simulink model "LaneChangePlanner"  (R2020b)
settings: Solver=FixedStepAuto  StartTime=0.0  StopTime=10.0  RelTol=1e-3
values from neighbouring files (symbols this model uses):
  minDistThreshold = 3.7    [setupscript.m]
  Ts = 0.1    [setupscript.m]
  v0_ego = egoCar.v0    [setupscript.m]
undefined symbols (not defined in the file or in its folder): planningHorizon
settings Model: Creator=The MathWorks, Inc.  LastModifiedBy=Milin
settings OptimizationCC: DefaultParameterBehavior=Inlined  EnhancedBackFolding=on  PassReuseOutputArgsAs=Individual arguments  ZeroExternalMemoryAtStartup=off  ZeroInternalMemoryAtStartup=off  OptimizeBlockOrder=speed  DifferentSizesBufferReuse=on  OptimizationCustomize=off  EfficientTunableParamExpr=on
settings DebuggingCC: ParameterTunabilityLossMsg=error
settings ModelReferenceCC: ModelReferenceNumInstancesAllowed=Single  PropagateVarSize=During execution
settings SFSimCC: MATLABDynamicMemAllocThreshold=0
settings RTWCC: Description=Embedded Coder  SystemTargetFile=ert.tlc  TemplateMakefile=ert_default_tmf
settings CodeAppCC: ForceParamTrailComments=on  IgnoreCustomStorageClasses=off  OperatorAnnotations=on  SimulinkDataObjDesc=on  SFDataObjDesc=on  InsertBlockDesc=on
settings ERTTargetCC: TargetLangStandard=C99 (ISO)  GenerateSampleERTMain=on  SupportVariableSizeSignals=on  InlinedParameterPlacement=NonHierarchical  ERTCustomFileTemplate=example_file_process.tlc

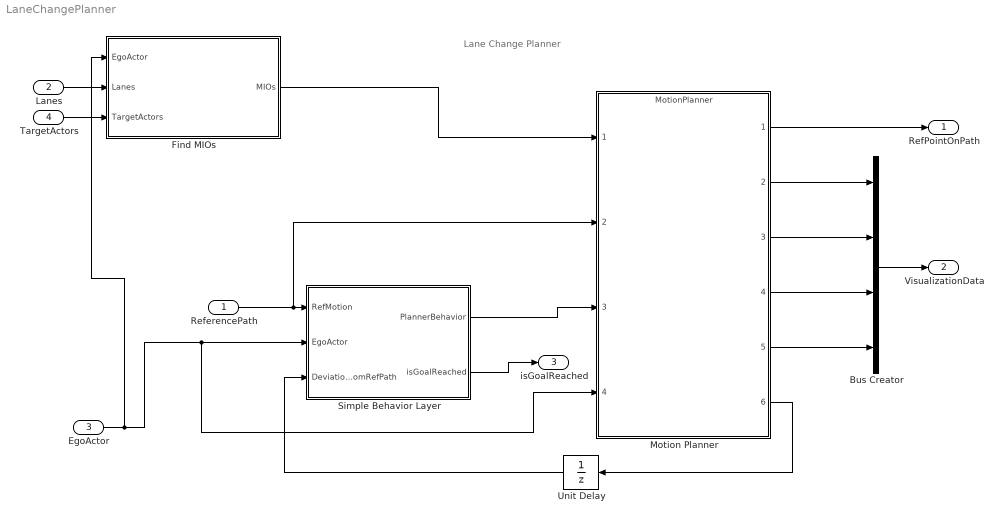
== system LaneChangePlanner ==
  note: Lane Change Planner
  ReferencePath : Inport
  Lanes : Inport  Port=2  OutDataTypeStr=Bus: BusLanes  BusOutputAsStruct=on
  EgoActor : Inport  Port=3  OutDataTypeStr=Bus: BusActors1Actors  BusOutputAsStruct=on
  TargetActors : Inport  Port=4  OutDataTypeStr=Bus: BusActors1  BusOutputAsStruct=on
  Bus Creator : BusCreator  Inputs=4  OutDataTypeStr=Bus: BusPlannerData
  Find MIOs : Subsystem
  Motion Planner : ModelReference  ModelNameDialog=MotionPlanner.slx  SimulationMode=Normal  CodeInterface=Top model  ModelReferenceVersion=1.92
  Simple Behavior Layer : Subsystem
  Unit Delay : UnitDelay  InitialCondition=-1.8000  SampleTime=-1  HasFrameUpgradeWarning=on
  RefPointOnPath : Outport  OutDataTypeStr=Bus: BusRefPointOnPath
  VisualizationData : Outport  Port=2  OutDataTypeStr=Bus: BusPlannerData
  isGoalReached : Outport  Port=3
  wires:
  Unit Delay/1 -> Simple Behavior Layer/3(DeviationFromRefPath)
  Motion Planner/6 -> Unit Delay/1
  Simple Behavior Layer/2(isGoalReached) -> isGoalReached/1
  Motion Planner/5 -> Bus Creator/4
  Bus Creator/1 -> VisualizationData/1
  Motion Planner/3 -> Bus Creator/2
  Motion Planner/4 -> Bus Creator/3
  Motion Planner/2 -> Bus Creator/1
  ReferencePath/1 -> Motion Planner/2, Simple Behavior Layer/1(RefMotion)
  Motion Planner/1 -> RefPointOnPath/1
  EgoActor/1 -> Find MIOs/1(EgoActor), Motion Planner/4, Simple Behavior Layer/2(EgoActor)
  Lanes/1 -> Find MIOs/2(Lanes)
  TargetActors/1 -> Find MIOs/3(TargetActors)
  Simple Behavior Layer/1(PlannerBehavior) -> Motion Planner/3
  Find MIOs/1(MIOs) -> Motion Planner/1

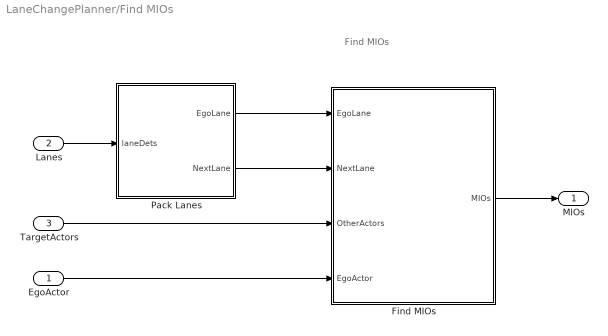
== system LaneChangePlanner/Find MIOs ==
  note: Find MIOs
  EgoActor : Inport
  Lanes : Inport  Port=2
  TargetActors : Inport  Port=3
  Find MIOs : MATLAB Function  TreatAsAtomicUnit=on
  Pack Lanes : MATLAB Function  TreatAsAtomicUnit=on
  MIOs : Outport
  wires:
  Pack Lanes/2(NextLane) -> Find MIOs/2(NextLane)
  Pack Lanes/1(EgoLane) -> Find MIOs/1(EgoLane)
  Lanes/1 -> Pack Lanes/1(laneDets)
  EgoActor/1 -> Find MIOs/4(EgoActor)
  TargetActors/1 -> Find MIOs/3(OtherActors)
  Find MIOs/1(MIOs) -> MIOs/1

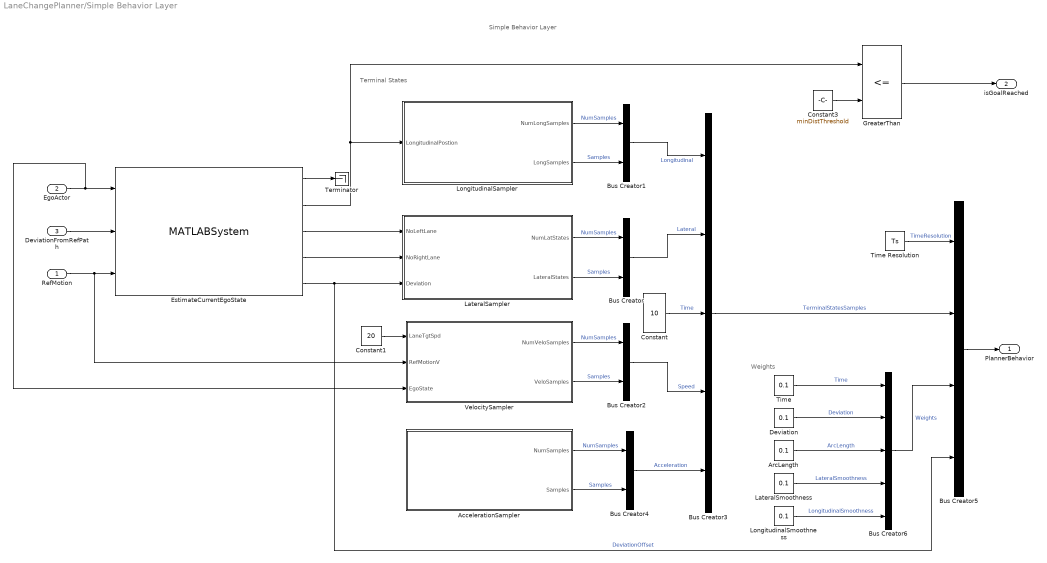
== system LaneChangePlanner/Simple Behavior Layer ==
  note: Weights
  note: Terminal States
  note: Simple Behavior Layer
  RefMotion : Inport
  EgoActor : Inport  Port=2
  DeviationFromRefPath : Inport  Port=3
  AccelerationSampler : Subsystem
  ArcLength : Constant  Value=0.1
  Bus Creator{,1..2,4} (4 alike) : BusCreator  Inputs=2
  Bus Creator3 : BusCreator  Inputs=5
  Bus Creator5 : BusCreator  Inputs=4  OutDataTypeStr=Bus: BusPlannerBehavior  NonVirtualBus=on
  Bus Creator6 : BusCreator  Inputs=5
  Constant : Constant  Value=10
  Constant1 : Constant  Value=20
  Constant3 : Constant  Value=minDistThreshold
  Deviation : Constant  Value=0.1
  EstimateCurrentEgoState : MATLABSystem  System=HelperEstimateCurrentEgoState  LaneWidth=laneWidth  EgoActorID=1  InitialDeviation=initialDeviation  InitialEgoLaneNumber=initialEgoLaneID  LaneType=laneType  SimulateUsing=Code generation
      mask Type: HelperEstimateCurrentEgoState
      mask Display:
      | disp('HelperEstimateCurrentEgoState');
      | port_label('input',1,'EgoActor');
      | port_label('input',2,'LateralDeviation');
      | port_label('input',3,'RefPath');
      | port_label('output',1,'LateralPosition');
      | port_label('output',2,'LongitudinalPosition');
      | port_label('output',3,'NoLeftLane');
      | port_label('output',4,'NoRightLane');
      | port_label('output',5,'DeviationOffset');
  GreaterThan : RelationalOperator  Operator=<=  OutDataTypeStr=boolean  RndMeth=Simplest
  LateralSampler : MATLAB Function  TreatAsAtomicUnit=on
  LateralSmoothness : Constant  Value=0.1
  LongitudinalSampler : MATLAB Function  TreatAsAtomicUnit=on  mask{planningHorizon=planningHorizon}
      mask prompts: planningHorizon "Planning Horizon"
  LongitudinalSmoothness : Constant  Value=0.1
  Terminator : Terminator
  Time : Constant  Value=0.1
  Time Resolution : Constant  Value=Ts
  VelocitySampler : MATLAB Function  TreatAsAtomicUnit=on  mask{egoSetVelocity=v0_ego}
      mask prompts: egoSetVelocity "Ego Set Velocity"
  PlannerBehavior : Outport  OutDataTypeStr=Bus: BusPlannerBehavior
  isGoalReached : Outport  Port=2
  wires:
  GreaterThan/1 -> isGoalReached/1
  VelocitySampler/2(VeloSamples) -> Bus Creator2/2  "Samples"
  RefMotion/1 -> EstimateCurrentEgoState/3, VelocitySampler/2(RefMotionV)
  EgoActor/1 -> EstimateCurrentEgoState/1, VelocitySampler/3(EgoState)
  Constant1/1 -> VelocitySampler/1(LaneTgtSpd)
  VelocitySampler/1(NumVeloSamples) -> Bus Creator2/1  "NumSamples"
  Constant3/1 -> GreaterThan/2
  Constant/1 -> Bus Creator3/3  "Time"
  EstimateCurrentEgoState/4 -> LateralSampler/2(NoRightLane)
  EstimateCurrentEgoState/3 -> LateralSampler/1(NoLeftLane)
  EstimateCurrentEgoState/2 -> GreaterThan/1, LongitudinalSampler/1(LongitudinalPostion)
  LongitudinalSampler/1(NumLongSamples) -> Bus Creator1/1  "NumSamples"
  LongitudinalSampler/2(LongSamples) -> Bus Creator1/2  "Samples"
  Bus Creator1/1 -> Bus Creator3/1  "Longitudinal"
  Bus Creator2/1 -> Bus Creator3/4  "Speed"
  EstimateCurrentEgoState/5 -> Bus Creator5/4, LateralSampler/3(Deviation)  "DeviationOffset"
  Bus Creator/1 -> Bus Creator3/2  "Lateral"
  LateralSampler/2(LateralStates) -> Bus Creator/2  "Samples"
  Bus Creator6/1 -> Bus Creator5/3  "Weights"
  Bus Creator3/1 -> Bus Creator5/2  "TerminalStatesSamples"
  Time Resolution/1 -> Bus Creator5/1  "TimeResolution"
  LongitudinalSmoothness/1 -> Bus Creator6/5  "LongitudinalSmoothness"
  LateralSmoothness/1 -> Bus Creator6/4  "LateralSmoothness"
  ArcLength/1 -> Bus Creator6/3  "ArcLength"
  Deviation/1 -> Bus Creator6/2  "Deviation"
  Time/1 -> Bus Creator6/1  "Time"
  Bus Creator4/1 -> Bus Creator3/5  "Acceleration"
  LateralSampler/1(NumLatStates) -> Bus Creator/1  "NumSamples"
  AccelerationSampler/2(Samples) -> Bus Creator4/2  "Samples"
  AccelerationSampler/1(NumSamples) -> Bus Creator4/1  "NumSamples"
  EstimateCurrentEgoState/1 -> Terminator/1
  Bus Creator5/1 -> PlannerBehavior/1
  DeviationFromRefPath/1 -> EstimateCurrentEgoState/2

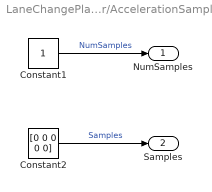
== system LaneChangePlanner/Simple Behavior Layer/AccelerationSampler ==
  Constant1 : Constant
  Constant2 : Constant  Value=[0 0 0 0 0]
  NumSamples : Outport
  Samples : Outport  Port=2
  wires:
  Constant1/1 -> NumSamples/1  "NumSamples"
  Constant2/1 -> Samples/1  "Samples"

== matlab function LaneChangePlanner/Find MIOs/Find MIOs ==
  data: EgoLane input; NextLane input; OtherActors input; EgoActor input; MIOs output Bus: BusMIOs
% Find front/rear MIO (Most Important Object) in the ego lane and front/rear
% MIOs in the left next lane.
function MIOs  = findMIOs( EgoLane, NextLane, OtherActors, EgoActor)

% If lane detection is not available, the ego car is assumed to be located
% in the middle of its lane. The lane width is assumed to be 3.6m, typical
% highway lane width.
laneWidth = 3.6;
halfLaneWidth = laneWidth/2;

% ego left lane detected?
if EgoLane.Left.Strength > 0.01 
    egoLeftLane = [EgoLane.Left.CurvatureDerivative/6,...
        EgoLane.Left.Curvature/2,...
        EgoLane.Left.HeadingAngle,...
        EgoLane.Left.LateralOffset];
else % ego left lane is not available
    egoLeftLane = single([0,0,0,halfLaneWidth]);
end
% ego right lane detected?
if EgoLane.Right.Strength > 0.01  
    egoRightLane = [EgoLane.Right.CurvatureDerivative/6,...
        EgoLane.Right.Curvature/2,...
        EgoLane.Right.HeadingAngle,...
        EgoLane.Right.LateralOffset];
else % ego right lane is not available
    egoRightLane = single([0,0,0,-halfLaneWidth]);    
end
% left next lane detected?
if NextLane.Left.Strength > 0.01 
    nextLeftLane = [NextLane.Left.CurvatureDerivative/6,...
        NextLane.Left.Curvature/2,...
        NextLane.Left.HeadingAngle,...
        NextLane.Left.LateralOffset];
else % left next lane is not available
    nextLeftLane = single([0,0,0,halfLaneWidth+laneWidth]);       
end
% right next lane detected?
if NextLane.Right.Strength > 0.01 
    nextRightLane = [NextLane.Right.CurvatureDerivative/6,...
        NextLane.Right.Curvature/2,...
        NextLane.Right.HeadingAngle,...
        NextLane.Right.LateralOffset];
else % right next lane is not available
    nextRightLane = single([0,0,0,halfLaneWidth+laneWidth]);       
end

% Initialize outputs and parameters
% Far enough forward so that no track is expected to exceed this distance
egoMaxX = cast(500, 'like', EgoActor.Position);
% Far enough forward so that no track is expected to exceed this distance
egoMinX = cast(-500, 'like', EgoActor.Position);  
% Far enough forward so that no track is expected to exceed this distance
leftNextMaxX = cast(500, 'like', EgoActor.Position);  
% Far enough rearward so that no track is expected to exceed this distance
leftNextMinX = cast(-500, 'like', EgoActor.Position);  
% Far enough forward so that no track is expected to exceed this distance
rightNextMaxX = cast(500, 'like', EgoActor.Position); 
% Far enough rearward so that no track is expected to exceed this distance
rightNextMinX = cast(-500, 'like', EgoActor.Position);

% initialize MIOs
EgoFront = struct(...
    'TrackIndex', uint32(0),...
    'Position', double([0 0]'), ...
    'Velocity', double([0 0]'), ...
    'RangeMagnitude', double(2000), ...  % default range = big number (ex. 2000)
    'VelocityMagnitude', double(0), ...
    'TTC', double(100));

EgoRear = struct(...
    'TrackIndex', uint32(0),...
    'Position', double([0 0]'), ...
    'Velocity', double([0 0]'), ...
    'RangeMagnitude', double(0), ...  
    'VelocityMagnitude', double(0), ...
    'TTC', double(0));

LeftFront = struct(...
    'TrackIndex', uint32(0),...
    'Position', double([0 0]'), ...
    'Velocity', double([0 0]'), ...
    'RangeMagnitude', double(0), ...
    'VelocityMagnitude', double(0), ...
    'TTC', double(0));

LeftRear = struct(...
    'TrackIndex', uint32(0),...
    'Position', double([0 0]'), ...
    'Velocity', double([0 0]'), ...
    'RangeMagnitude', double(0), ...
    'VelocityMagnitude', double(0), ...
    'TTC', double(0));

RightFront = struct(...
    'TrackIndex', uint32(0),...
    'Position', double([0 0]'), ...
    'Velocity', double([0 0]'), ...
    'RangeMagnitude', double(0), ...
    'VelocityMagnitude', double(0), ...
    'TTC', double(0));

RightRear = struct(...
    'TrackIndex', uint32(0),...
    'Position', double([0 0]'), ...
    'Velocity', double([0 0]'), ...
    'RangeMagnitude', double(0), ...
    'VelocityMagnitude', double(0), ...
    'TTC', double(0));
MIOs = struct(...
    'NumMIOs',uint32(0),...
    'MIOObjects', repmat(RightFront,6,1));

for i = 1:OtherActors.NumActors
    position = OtherActors.Actors(i).Position;
    % Longitudinal position of the target vehicle relative to ego
    x = position(1);
    % Lateral position of the target vehicle relative to ego
    y = position(2); 
    
    % lateral position of left ego lane   
    yEgoLaneLeft  = polyval(egoLeftLane,x); 
     % lateral position of right ego lane
    yEgoLaneRight = polyval(egoRightLane,x);
    
    % Check for ego front MIO
    if laneWidth < x && x < egoMaxX
        % Check for the target vehicles lane. Is it with in  the ego lane?
        if (yEgoLaneRight <= y) && (y <= yEgoLaneLeft) 
            egoMaxX = x;
            % save track index for frontEgo MIO
            EgoFront.TrackIndex = uint32(i);
        end
    end   
    % Check of ego rear MIO
    if egoMinX < x && x < -1        
        if (yEgoLaneRight <= y) && (y <= yEgoLaneLeft)
            egoMinX = x;
            % save track index for rearEgo MIO
            EgoRear.TrackIndex = uint32(i); 
        end
    end
    % Check for next lane
    if NextLane.Left.Strength > 0.01 
        % left next lane
        yNextLaneLeft = polyval(nextLeftLane,x);  
        % right = ego left lane
        yNextLaneRight = polyval(egoLeftLane,x); 
        
        % Check for left front MIO
        if 0 < x && x < leftNextMaxX            
            if (yNextLaneRight <= y) && (y <= yNextLaneLeft) 
                leftNextMaxX = x;
                % save track index for nextFront MIO
                LeftFront.TrackIndex = uint32(i); 
            end
        end
        % Check for left rear MIO
        if leftNextMinX < x && x < 0            
            if (yNextLaneRight <= y) && (y <= yNextLaneLeft) 
                leftNextMinX = x;
                % save track index for nextRear MIO
                LeftRear.TrackIndex = uint32(i); 
            end
        end
    end
    % left next lane detected?
    if NextLane.Right.Strength > 0.01 
        % left = ego right lane
        yNextLaneLeft = polyval(egoRightLane,x); 
        % right next lane
        yNextLaneRight = polyval(nextRightLane,x);  
        
        % Check for Ego right front MIO
        if 0 < x && x < rightNextMaxX            
            if (yNextLaneRight <= y) && (y <= yNextLaneLeft) 
                rightNextMaxX = x;
                % save track index for nextFront MIO
                RightFront.TrackIndex = uint32(i); 
            end
        end
        % Check for Ego right rear MIO
        if rightNextMinX < x && x < 0            
            if (yNextLaneRight <= y) && (y <= yNextLaneLeft) 
                rightNextMinX = x;
                % save track index for nextRear MIO
                RightRear.TrackIndex = uint32(i); 
            end
        end
    end    
end
% egoFront MIO detected?
if EgoFront.TrackIndex > 0 
    EgoFront.Position = OtherActors.Actors(EgoFront.TrackIndex).Position(1:2)';
    EgoFront.Velocity = OtherActors.Actors(EgoFront.TrackIndex).Velocity(1:2)';
    [EgoFront.RangeMagnitude, EgoFront.VelocityMagnitude, EgoFront.TTC] = ...
        calculateTTC(EgoFront.Position,EgoFront.Velocity);    
end
% egoRear MIO detected?
if EgoRear.TrackIndex > 0 
    EgoRear.Position = OtherActors.Actors(EgoRear.TrackIndex).Position(1:2)';
    EgoRear.Velocity = OtherActors.Actors(EgoRear.TrackIndex).Velocity(1:2)';
    [EgoRear.RangeMagnitude, EgoRear.VelocityMagnitude, EgoRear.TTC] = ...
        calculateTTC(EgoRear.Position,EgoRear.Velocity);    
end
% leftFront MIO detected?
if LeftFront.TrackIndex > 0 
    LeftFront.Position = OtherActors.Actors(LeftFront.TrackIndex).Position(1:2)';
    LeftFront.Velocity = OtherActors.Actors(LeftFront.TrackIndex).Velocity(1:2)';  
    [LeftFront.RangeMagnitude, LeftFront.VelocityMagnitude, LeftFront.TTC] = ...
        calculateTTC(LeftFront.Position,LeftFront.Velocity);    
end
% leftRear MIO detected? 
if LeftRear.TrackIndex > 0 
    LeftRear.Position = OtherActors.Actors(LeftRear.TrackIndex).Position(1:2)';
    LeftRear.Velocity = OtherActors.Actors(LeftRear.TrackIndex).Velocity(1:2)';    
    [LeftRear.RangeMagnitude, LeftRear.VelocityMagnitude, LeftRear.TTC] = ...
        calculateTTC(LeftRear.Position,LeftRear.Velocity);      
end
% dightFront MIO detected?
if RightFront.TrackIndex > 0 
    RightFront.Position = OtherActors.Actors(RightFront.TrackIndex).Position(1:2)';
    RightFront.Velocity = OtherActors.Actors(RightFront.TrackIndex).Velocity(1:2)';    
    [RightFront.RangeMagnitude, RightFront.VelocityMagnitude, RightFront.TTC] = ...
        calculateTTC(RightFront.Position,RightFront.Velocity);    
end
% rightRear MIO detected?
if RightRear.TrackIndex > 0  
    RightRear.Position = OtherActors.Actors(RightRear.TrackIndex).Position(1:2)';
    RightRear.Velocity = OtherActors.Actors(RightRear.TrackIndex).Velocity(1:2)';     
    [RightRear.RangeMagnitude, RightRear.VelocityMagnitude, RightRear.TTC] = ...
        calculateTTC(RightRear.Position,RightRear.Velocity);      
end
MIOs.NumMIOs = uint32(6);
MIOs.MIOObjects(1,1) = EgoFront;
MIOs.MIOObjects(2,1) = EgoRear;
MIOs.MIOObjects(3,1) = LeftFront;
MIOs.MIOObjects(4,1) = LeftRear;
MIOs.MIOObjects(5,1) = RightFront;
MIOs.MIOObjects(6,1) = RightRear;
end

% calculate magnitude of range and velocity, Time-to-contact (TTC) for MIO
function [RangeMagnitude,VelocityMagnitude,ttc] = calculateTTC(position,velocity)

[RangeAngle,RangeMagnitude] = cart2pol(position(1),position(2));
[VelocityAngle,vel] = cart2pol(velocity(1),velocity(2));

VelocityMagnitude = vel * cos(VelocityAngle-RangeAngle);
% limit speed to +/-0.1 m/s for ttc calculation
if abs(VelocityMagnitude)<0.1 
    if VelocityMagnitude>=0
        vel(:) = 0.1;
    else
        vel(:) = -0.1;
    end
else
    vel(:) = VelocityMagnitude;
end
% Time-To-Contact (sec)
ttc = RangeMagnitude/vel;
        
end

== matlab function LaneChangePlanner/Find MIOs/Pack Lanes ==
  data: laneDets input Bus: BusLanes; EgoLane output Bus: LaneSensor; NextLane output Bus: LaneSensor
%% packLanes
% This function extracts ego and next left lanes and pack them with
%  BusLaneSensor
function [EgoLane,NextLane] = packLanes(laneDets)

numLanes = laneDets.NumLaneBoundaries;
lanes = laneDets.LaneBoundaries;

% read lateral offset for all lanes
offset = zeros(numLanes,1);
for i = 1:numLanes
    offset(i) = lanes(i).LateralOffset;
end

% create dummy lane with zero strength
dummyLane = struct(...
    'Curvature',single(0),...
    'CurvatureDerivative', single(0), ...
    'HeadingAngle', single(0), ...
    'LateralOffset', single(0), ...
    'Strength', single(0));

% sort the lateral offset
rb = sort(offset(offset<=0),'descend');  % right lanes 
lb = sort(offset(offset>0),'ascend');    % left lane

if length(lb)>=2 % both left ego and next lanes exist?
    egoLeftIndx = searchIndx(offset, numLanes, lb(1)); % index for ego left lane
    EgoLane.Left = getLaneParameters(lanes(egoLeftIndx));

    nextLeftIndx = searchIndx(offset, numLanes, lb(2)); % index for left next lane  
    NextLane.Left = getLaneParameters(lanes(nextLeftIndx));
elseif length(lb)==1 % no left next lane, only left ego lane?
    egoLeftIndx = searchIndx(offset, numLanes, lb(1));  % index for left ego lane 
    EgoLane.Left = getLaneParameters(lanes(egoLeftIndx));
    
    NextLane.Left = dummyLane; % no left next lane
else % no left lanes
    EgoLane.Left = dummyLane;  % no left ego lane
    NextLane.Left = dummyLane; % no left next lane  
end

if length(rb)>=2 % both right ego and next lanes exist?
    egoRightIndx = searchIndx(offset, numLanes, rb(1));  % index for right ego lane   
    EgoLane.Right = getLaneParameters(lanes(egoRightIndx));

    nextRightIndx = searchIndx(offset, numLanes, rb(2)); % index for right next lane      
    NextLane.Right = getLaneParameters(lanes(nextRightIndx));
elseif length(rb)==1 % no right next lane, only right ego lane?
    egoRightIndx = searchIndx(offset, numLanes, rb(1));  % index for right ego lane   
    EgoLane.Right = getLaneParameters(lanes(egoRightIndx));
    
    NextLane.Right = dummyLane; % no right next lane
else % no right lanes
    EgoLane.Right = dummyLane;  % no right ego lane
    NextLane.Right = dummyLane; % no right next lane    
end

end
% Search for next index
function indx = searchIndx(offset, num, val)

indx = 0;
for i = 1:num
    if offset(i) == val
        indx = i;
        return;
    end
end

end

% read laneBoundaries and convert units from deg to rad
function laneSensor = getLaneParameters(LaneBoundaries)

laneSensor.Curvature = single(deg2rad(LaneBoundaries.Curvature));
laneSensor.CurvatureDerivative = single(deg2rad(LaneBoundaries.CurvatureDerivative));
laneSensor.HeadingAngle = single(deg2rad(LaneBoundaries.HeadingAngle));
laneSensor.LateralOffset = single(LaneBoundaries.LateralOffset);
laneSensor.Strength = single(LaneBoundaries.Strength);

end

== matlab function LaneChangePlanner/Simple Behavior Layer/LongitudinalSampler ==
  data: LongitudinalPostion input; NumLongSamples output; LongSamples output; planningHorizon parameter
%% LongitudinalSampler 
% LongitudinalSampler samples the possible longitudinal terminal state for
% the planner
function [NumLongSamples,LongSamples] = LongitudinalSampler(LongitudinalPostion,...
                                                            planningHorizon)
LongSamples = zeros(1,5);

% Default offset or stoppoing distance from the goal point is 1 meter
offsetDistance = 1;
% Number of longitudinal sample is one.
NumLongSamples = 1;

% Check the distance to the goal point.
% Update the LongSamples based on the distance to the goal point
if(LongitudinalPostion <= planningHorizon)
    LongSamples(1,1) = LongitudinalPostion - offsetDistance;
else
    LongSamples(1,1) = planningHorizon;
end
end

== matlab function LaneChangePlanner/Simple Behavior Layer/LateralSampler ==
  data: NoLeftLane input; NumLatStates output; NoRightLane input; Deviation input; LateralStates output
%%LateralSampler 
% LateralSampler samples the possible lateral terminal state for
% the planner
function [NumLatStates, LateralStates] = LateralSampler(NoLeftLane,...
                                                        NoRightLane,...
                                                        Deviation)
%LateralSampler function updates the laterla states by checking the existance
% of the right and left lanes from the current ego lane.
LateralStates = zeros(1,5);
% Assumed lane width is 3.6 meters
LaneWidth = 3.6;

% Update LateralStates by checking the existence of adjacent lanes.
if ~NoLeftLane && ~NoRightLane
    NumLatStates = 3;
    LateralStates(1,1:NumLatStates) = [Deviation + LaneWidth, Deviation, Deviation - LaneWidth];
elseif NoLeftLane
    NumLatStates = 2;
    LateralStates(1,1:NumLatStates) = [Deviation - LaneWidth, Deviation];
elseif NoRightLane
    NumLatStates = 2;
    LateralStates(1,1:NumLatStates) = [Deviation + LaneWidth, Deviation];
else
    NumLatStates = 1;
end

end

== matlab function LaneChangePlanner/Simple Behavior Layer/VelocitySampler ==
  data: LaneTgtSpd input; NumVeloSamples output; RefMotionV input; EgoState input; VeloSamples output; egoSetVelocity parameter
%%VelocitySampler 
% VelocitySampler samples the possible velocity terminal state for
% the planner
function [NumVeloSamples,VeloSamples] = VelocitySampler(LaneTgtSpd,...
                                                        RefMotionV,...
                                                        EgoState,...
                                                        egoSetVelocity)
% Currently this function is a place holder. This function is intended to 
% consider lane speed velocity profile generated for the reference path
% while generating trjectory
VeloSamples = zeros(1,5);
NumVeloSamples = 1;

VeloSamples(1,1) = egoSetVelocity;
end
